simulink library "PTOSim_Lib"  (R2014a)
settings: Solver=ode45  StartTime=0.0  StopTime=10.0  RelTol=1e-3
undefined symbols (not defined in the file): alpha, Amax, Amin, Ap, Beta_e, bf, bg, Cd, D, driveEff, J, k1, k2, omegaBase, omegaInit, pAeq, pAi, pAupper_limit, pBeq, pBi, pBupper_limit, pCprecharge, pDprecharge, pMax, pMin, rho, TgenBase, tot, VC0, VCeq, VD0, VDeq, Vo
settings Model: ForwardingTableString=||__slOldName__||Y:\MATLAB\PTO-Sim\Source\lib||__slNewName__||Y:\MATLAB\PTO-Sim\PassiveHydraulicPTO  Creator=sor  LastModifiedBy=sor

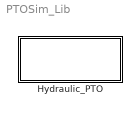
== system PTOSim_Lib ==
  Hydraulic_PTO : Subsystem  RequirementInfo={} %GIDa_f12a42eb_b9cb_4818_b573_b7dee4183a3b

== system PTOSim_Lib/Hydraulic_PTO ==
  Accumulator : Subsystem  Variant=on  mask{pto=0}
      mask prompts: pto "PTO Name"
  Gen Drive Efficiency : Subsystem  mask{pto=0}
      mask prompts: pto "PTO Name"
  "Motor " : Subsystem  mask{pto=0}
      mask prompts: pto "PTO Name"
  "Piston " : Subsystem  mask{pto=0}
      mask prompts: pto "PTO Name"
  Rectified Valve : Subsystem  mask{pto=0}
      mask prompts: pto "PTO Name"

== system PTOSim_Lib/Hydraulic_PTO/Accumulator ==
  note: 1) Only subsystems can be added as variant choices at this level
      | 2) Blocks cannot be connected at this level as connectivity is
      | automatically determined at simulation, based on the active variant
  Vdot : Inport
  Vdotm : Inport  Port=2
  High Pressure Accumulator : Subsystem  VariantControl=Variant
  Low Pressure Accumulator : Subsystem  VariantControl=Variant1
  Pressure : Outport

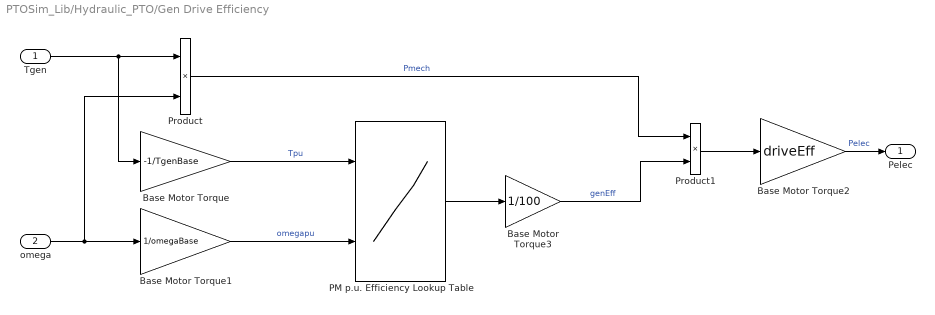
== system PTOSim_Lib/Hydraulic_PTO/Gen Drive Efficiency ==
  Tgen : Inport
  omega : Inport  Port=2
  Base Motor Torque : Gain  Gain=-1/TgenBase
  Base Motor Torque1 : Gain  Gain=1/omegaBase
  Base Motor Torque2 : Gain  Gain=driveEff
  Base Motor Torque3 : Gain  Gain=1/100
  PM p.u. Efficiency Lookup Table : Lookup_n-D  BreakpointsForDimension1=tot.Tpu(:,1)  BreakpointsForDimension2=tot.omegapu(1,:)  Table=tot.eff  InterpMethod=Flat  InputSameDT=on
  Product : Product  RndMeth=Zero
  Product1 : Product  RndMeth=Zero
  Pelec : Outport
  wires:
  Base Motor Torque2/1 -> Pelec/1  "Pelec"
  Product1/1 -> Base Motor Torque2/1
  Product/1 -> Product1/1  "Pmech"
  Base Motor Torque3/1 -> Product1/2  "genEff"
  PM p.u. Efficiency Lookup Table/1 -> Base Motor Torque3/1
  omega/1 -> Product/2, Base Motor Torque1/1
  Base Motor Torque1/1 -> PM p.u. Efficiency Lookup Table/2  "omegapu"
  Tgen/1 -> Base Motor Torque/1, Product/1
  Base Motor Torque/1 -> PM p.u. Efficiency Lookup Table/1  "Tpu"

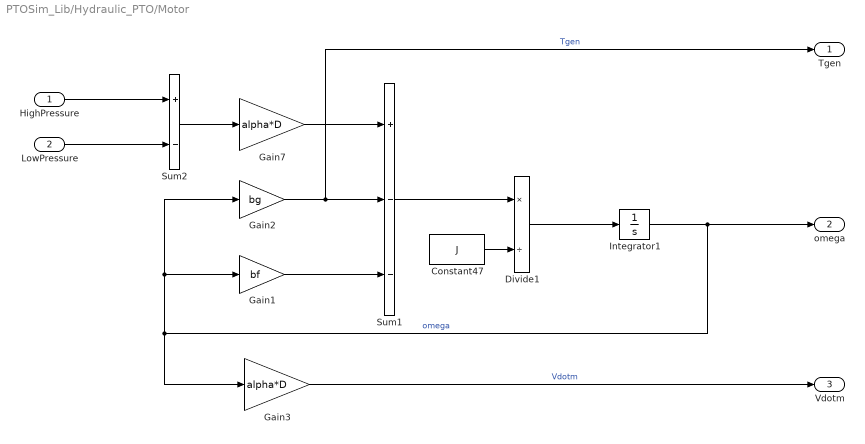
== system PTOSim_Lib/Hydraulic_PTO/Motor  ==
  HighPressure : Inport
  LowPressure : Inport  Port=2
  Constant47 : Constant  Value=J
  Divide1 : Product  Inputs=*/
  Gain1 : Gain  Gain=bf
  Gain2 : Gain  Gain=bg
  Gain3 : Gain  Gain=alpha*D
  Gain7 : Gain  Gain=alpha*D
  Integrator1 : Integrator  InitialCondition=omegaInit
  Sum1 : Sum  Inputs=+--
  Sum2 : Sum  Inputs=+-
  Tgen : Outport
  omega : Outport  Port=2
  Vdotm : Outport  Port=3
  wires:
  Gain7/1 -> Sum1/1
  Gain2/1 -> Tgen/1, Sum1/2  "Tgen"
  Gain1/1 -> Sum1/3
  Sum1/1 -> Divide1/1
  Constant47/1 -> Divide1/2
  Divide1/1 -> Integrator1/1
  Integrator1/1 -> omega/1, Gain3/1, Gain1/1, Gain2/1  "omega"
  Gain3/1 -> Vdotm/1  "Vdotm"
  HighPressure/1 -> Sum2/1
  LowPressure/1 -> Sum2/2
  Sum2/1 -> Gain7/1

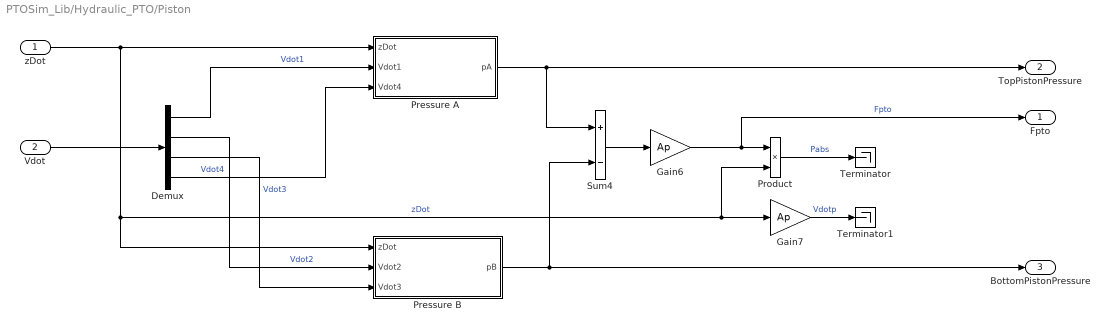
== system PTOSim_Lib/Hydraulic_PTO/Piston  ==
  zDot : Inport
  Vdot : Inport  Port=2
  Demux : Demux
  Gain6 : Gain  Gain=Ap
  Gain7 : Gain  Gain=Ap
  Pressure A : Subsystem
  Pressure B : Subsystem
  Product : Product
  Sum4 : Sum  Inputs=+-
  Terminator : Terminator
  Terminator1 : Terminator
  Fpto : Outport
  TopPistonPressure : Outport  Port=2
  BottomPistonPressure : Outport  Port=3
  wires:
  Pressure A/1(pA) -> Sum4/1, TopPistonPressure/1
  Pressure B/1(pB) -> BottomPistonPressure/1, Sum4/2
  Gain7/1 -> Terminator1/1  "Vdotp"
  Gain6/1 -> Fpto/1, Product/1  "Fpto"
  Product/1 -> Terminator/1  "Pabs"
  Vdot/1 -> Demux/1
  zDot/1 -> Gain7/1, Product/2, Pressure B/1(zDot), Pressure A/1(zDot)  "zDot"
  Demux/1 -> Pressure A/2(Vdot1)  "Vdot1"
  Demux/2 -> Pressure B/2(Vdot2)  "Vdot2"
  Demux/3 -> Pressure B/3(Vdot3)  "Vdot3"
  Demux/4 -> Pressure A/3(Vdot4)  "Vdot4"
  Sum4/1 -> Gain6/1

== system PTOSim_Lib/Hydraulic_PTO/Rectified Valve ==
  TopPistonPressure : Inport
  BottomPistonPressure : Inport  Port=2
  HighPressure : Inport  Port=3
  LowPressure : Inport  Port=4
  Bus Creator : BusCreator
  Subsystem : Subsystem
  Subsystem1 : Subsystem
  Subsystem2 : Subsystem
  Subsystem3 : Subsystem
  Vdot : Outport
  wires:
  TopPistonPressure/1 -> Subsystem3/2(pA), Subsystem/1(pA)
  BottomPistonPressure/1 -> Subsystem2/2(pB), Subsystem1/1(pB)
  HighPressure/1 -> Subsystem1/2(pC), Subsystem/2(pC)
  LowPressure/1 -> Subsystem3/1(pD), Subsystem2/1(pD)
  Subsystem3/1(Vdot4) -> Bus Creator/4  "Vdot4"
  Subsystem2/1(Vdot3) -> Bus Creator/3  "Vdot3"
  Subsystem1/1(Vdot2) -> Bus Creator/2  "Vdot2"
  Subsystem/1(Vdot1) -> Bus Creator/1  "Vdot1"
  Bus Creator/1 -> Vdot/1

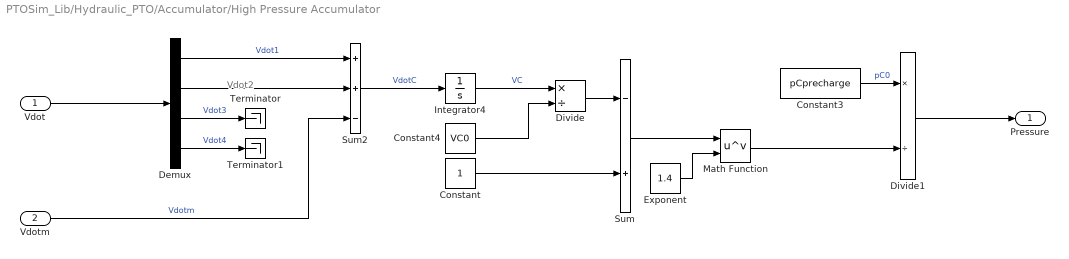
== system PTOSim_Lib/Hydraulic_PTO/Accumulator/High Pressure Accumulator ==
  note: Vdot2
  Vdot : Inport
  Vdotm : Inport  Port=2
  Constant : Constant
  Constant3 : Constant  Value=pCprecharge
  Constant4 : Constant  Value=VC0
  Demux : Demux
  Divide : Product  Inputs=*/
  Divide1 : Product  Inputs=*/
  Exponent : Constant  Value=1.4
  Integrator4 : Integrator  InitialCondition=VCeq
  Math Function : Math  Operator=pow  SaturateOnIntegerOverflow=on
  Sum : Sum  Inputs=-+
  Sum2 : Sum  Inputs=++-
  Terminator : Terminator
  Terminator1 : Terminator
  Pressure : Outport
  wires:
  Sum2/1 -> Integrator4/1  "VdotC"
  Integrator4/1 -> Divide/1  "VC"
  Constant4/1 -> Divide/2
  Constant/1 -> Sum/2
  Divide/1 -> Sum/1
  Exponent/1 -> Math Function/2
  Sum/1 -> Math Function/1
  Math Function/1 -> Divide1/2
  Constant3/1 -> Divide1/1  "pC0"
  Divide1/1 -> Pressure/1
  Vdot/1 -> Demux/1
  Demux/3 -> Terminator/1  "Vdot3"
  Demux/4 -> Terminator1/1  "Vdot4"
  Demux/1 -> Sum2/1  "Vdot1"
  Demux/2 -> Sum2/2
  Vdotm/1 -> Sum2/3  "Vdotm"

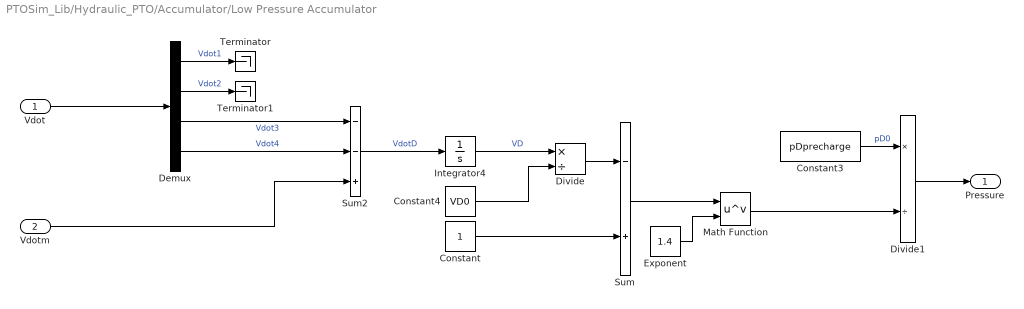
== system PTOSim_Lib/Hydraulic_PTO/Accumulator/Low Pressure Accumulator ==
  Vdot : Inport
  Vdotm : Inport  Port=2
  Constant : Constant
  Constant3 : Constant  Value=pDprecharge
  Constant4 : Constant  Value=VD0
  Demux : Demux
  Divide : Product  Inputs=*/
  Divide1 : Product  Inputs=*/
  Exponent : Constant  Value=1.4
  Integrator4 : Integrator  InitialCondition=VDeq
  Math Function : Math  Operator=pow  SaturateOnIntegerOverflow=on
  Sum : Sum  Inputs=-+
  Sum2 : Sum  Inputs=--+
  Terminator : Terminator
  Terminator1 : Terminator
  Pressure : Outport
  wires:
  Sum2/1 -> Integrator4/1  "VdotD"
  Integrator4/1 -> Divide/1  "VD"
  Constant4/1 -> Divide/2
  Constant/1 -> Sum/2
  Divide/1 -> Sum/1
  Exponent/1 -> Math Function/2
  Sum/1 -> Math Function/1
  Math Function/1 -> Divide1/2
  Constant3/1 -> Divide1/1  "pD0"
  Divide1/1 -> Pressure/1
  Vdot/1 -> Demux/1
  Demux/3 -> Sum2/1  "Vdot3"
  Demux/4 -> Sum2/2  "Vdot4"
  Vdotm/1 -> Sum2/3
  Demux/1 -> Terminator/1  "Vdot1"
  Demux/2 -> Terminator1/1  "Vdot2"

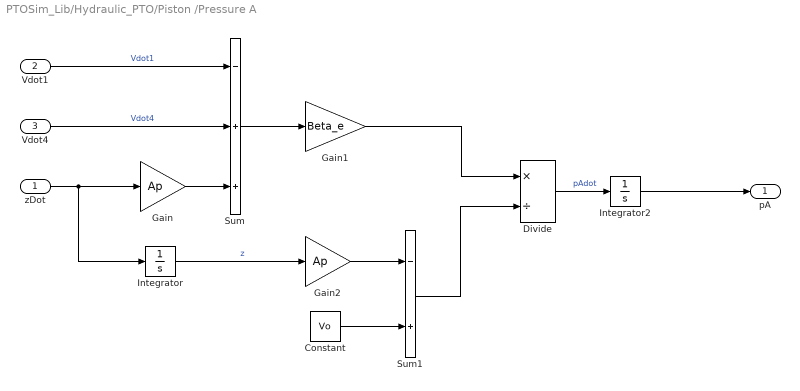
== system PTOSim_Lib/Hydraulic_PTO/Piston /Pressure A ==
  zDot : Inport
  Vdot1 : Inport  Port=2
  Vdot4 : Inport  Port=3
  Constant : Constant  Value=Vo
  Divide : Product  Inputs=*/
  Gain : Gain  Gain=Ap
  Gain1 : Gain  Gain=Beta_e
  Gain2 : Gain  Gain=Ap
  Integrator : Integrator
  Integrator2 : Integrator  InitialCondition=pAi  UpperSaturationLimit=pAupper_limit  LowerSaturationLimit=pAeq
  Sum : Sum  Inputs=-++
  Sum1 : Sum  Inputs=-+
  pA : Outport
  wires:
  Gain/1 -> Sum/3
  Sum/1 -> Gain1/1
  zDot/1 -> Integrator/1, Gain/1
  Integrator/1 -> Gain2/1  "z"
  Gain2/1 -> Sum1/1
  Constant/1 -> Sum1/2
  Gain1/1 -> Divide/1
  Sum1/1 -> Divide/2
  Vdot1/1 -> Sum/1  "Vdot1"
  Divide/1 -> Integrator2/1  "pAdot"
  Vdot4/1 -> Sum/2  "Vdot4"
  Integrator2/1 -> pA/1

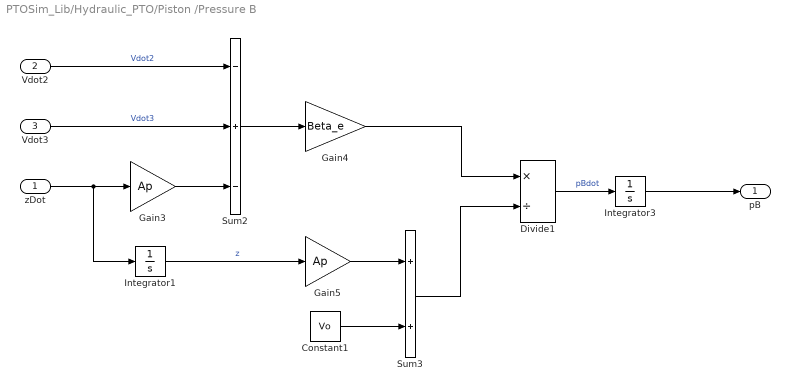
== system PTOSim_Lib/Hydraulic_PTO/Piston /Pressure B ==
  zDot : Inport
  Vdot2 : Inport  Port=2
  Vdot3 : Inport  Port=3
  Constant1 : Constant  Value=Vo
  Divide1 : Product  Inputs=*/
  Gain3 : Gain  Gain=Ap
  Gain4 : Gain  Gain=Beta_e
  Gain5 : Gain  Gain=Ap
  Integrator1 : Integrator
  Integrator3 : Integrator  InitialCondition=pBi  UpperSaturationLimit=pBupper_limit  LowerSaturationLimit=pBeq
  Sum2 : Sum  Inputs=-+-
  Sum3 : Sum
  pB : Outport
  wires:
  Gain3/1 -> Sum2/3
  Sum2/1 -> Gain4/1
  zDot/1 -> Integrator1/1, Gain3/1
  Integrator1/1 -> Gain5/1  "z"
  Gain5/1 -> Sum3/1
  Constant1/1 -> Sum3/2
  Gain4/1 -> Divide1/1
  Sum3/1 -> Divide1/2
  Divide1/1 -> Integrator3/1  "pBdot"
  Vdot2/1 -> Sum2/1  "Vdot2"
  Vdot3/1 -> Sum2/2  "Vdot3"
  Integrator3/1 -> pB/1

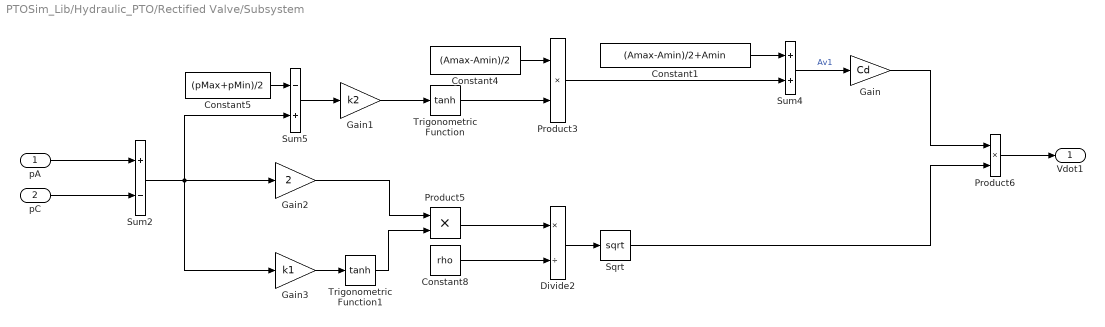
== system PTOSim_Lib/Hydraulic_PTO/Rectified Valve/Subsystem ==
  pA : Inport
  pC : Inport  Port=2
  Constant1 : Constant  Value=(Amax-Amin)/2+Amin
  Constant4 : Constant  Value=(Amax-Amin)/2
  Constant5 : Constant  Value=(pMax+pMin)/2
  Constant8 : Constant  Value=rho
  Divide2 : Product  Inputs=*/
  Gain : Gain  Gain=Cd
  Gain1 : Gain  Gain=k2
  Gain2 : Gain  Gain=2
  Gain3 : Gain  Gain=k1
  Product3 : Product
  Product5 : Product
  Product6 : Product
  Sqrt : Sqrt  SaturateOnIntegerOverflow=on
  Sum2 : Sum  Inputs=+-
  Sum4 : Sum
  Sum5 : Sum  Inputs=-+
  Trigonometric Function : Trigonometry  Operator=tanh
  Trigonometric Function1 : Trigonometry  Operator=tanh
  Vdot1 : Outport
  wires:
  Gain1/1 -> Trigonometric Function/1
  Trigonometric Function/1 -> Product3/2
  Product3/1 -> Sum4/2
  Sum5/1 -> Gain1/1
  Sum4/1 -> Gain/1  "Av1"
  Gain3/1 -> Trigonometric Function1/1
  Gain2/1 -> Product5/1
  Trigonometric Function1/1 -> Product5/2
  Sqrt/1 -> Product6/2
  Gain/1 -> Product6/1
  Constant8/1 -> Divide2/2
  Product5/1 -> Divide2/1
  Divide2/1 -> Sqrt/1
  pA/1 -> Sum2/1
  pC/1 -> Sum2/2
  Product6/1 -> Vdot1/1
  Constant4/1 -> Product3/1
  Constant5/1 -> Sum5/1
  Constant1/1 -> Sum4/1
  Sum2/1 -> Gain3/1, Sum5/2, Gain2/1

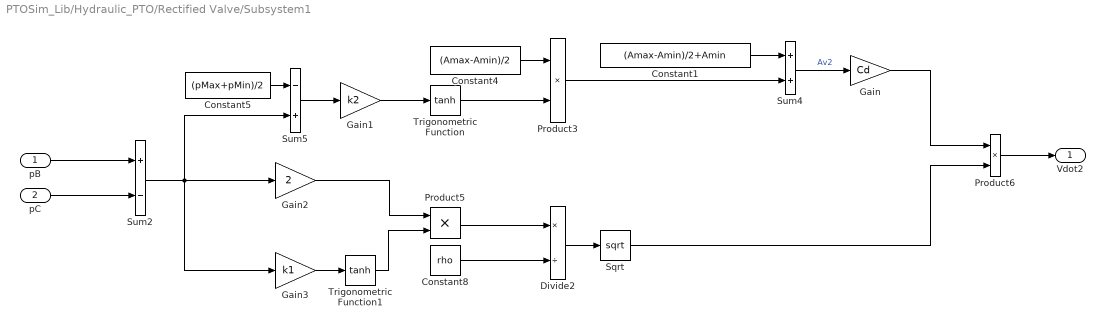
== system PTOSim_Lib/Hydraulic_PTO/Rectified Valve/Subsystem1 ==
  pB : Inport
  pC : Inport  Port=2
  Constant1 : Constant  Value=(Amax-Amin)/2+Amin
  Constant4 : Constant  Value=(Amax-Amin)/2
  Constant5 : Constant  Value=(pMax+pMin)/2
  Constant8 : Constant  Value=rho
  Divide2 : Product  Inputs=*/
  Gain : Gain  Gain=Cd
  Gain1 : Gain  Gain=k2
  Gain2 : Gain  Gain=2
  Gain3 : Gain  Gain=k1
  Product3 : Product
  Product5 : Product
  Product6 : Product
  Sqrt : Sqrt  SaturateOnIntegerOverflow=on
  Sum2 : Sum  Inputs=+-
  Sum4 : Sum
  Sum5 : Sum  Inputs=-+
  Trigonometric Function : Trigonometry  Operator=tanh
  Trigonometric Function1 : Trigonometry  Operator=tanh
  Vdot2 : Outport
  wires:
  Gain1/1 -> Trigonometric Function/1
  Trigonometric Function/1 -> Product3/2
  Product3/1 -> Sum4/2
  Sum5/1 -> Gain1/1
  Sum4/1 -> Gain/1  "Av2"
  Gain3/1 -> Trigonometric Function1/1
  Gain2/1 -> Product5/1
  Trigonometric Function1/1 -> Product5/2
  Sqrt/1 -> Product6/2
  Gain/1 -> Product6/1
  Constant8/1 -> Divide2/2
  Product5/1 -> Divide2/1
  Divide2/1 -> Sqrt/1
  pB/1 -> Sum2/1
  pC/1 -> Sum2/2
  Product6/1 -> Vdot2/1
  Constant4/1 -> Product3/1
  Constant5/1 -> Sum5/1
  Constant1/1 -> Sum4/1
  Sum2/1 -> Gain3/1, Sum5/2, Gain2/1

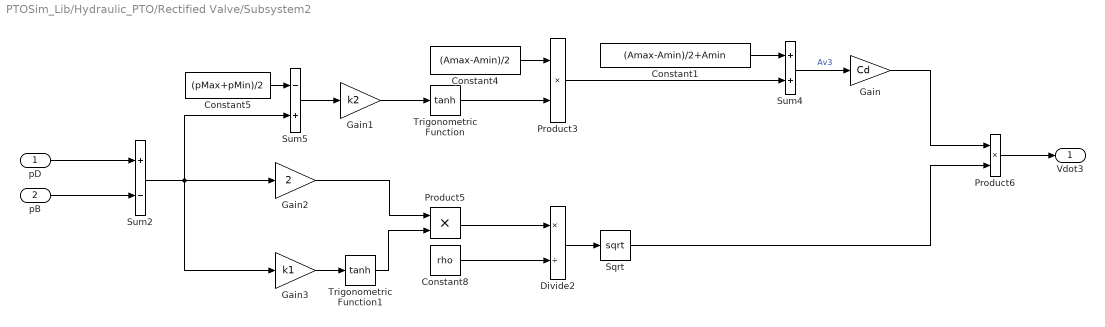
== system PTOSim_Lib/Hydraulic_PTO/Rectified Valve/Subsystem2 ==
  pD : Inport
  pB : Inport  Port=2
  Constant1 : Constant  Value=(Amax-Amin)/2+Amin
  Constant4 : Constant  Value=(Amax-Amin)/2
  Constant5 : Constant  Value=(pMax+pMin)/2
  Constant8 : Constant  Value=rho
  Divide2 : Product  Inputs=*/
  Gain : Gain  Gain=Cd
  Gain1 : Gain  Gain=k2
  Gain2 : Gain  Gain=2
  Gain3 : Gain  Gain=k1
  Product3 : Product
  Product5 : Product
  Product6 : Product
  Sqrt : Sqrt  SaturateOnIntegerOverflow=on
  Sum2 : Sum  Inputs=+-
  Sum4 : Sum
  Sum5 : Sum  Inputs=-+
  Trigonometric Function : Trigonometry  Operator=tanh
  Trigonometric Function1 : Trigonometry  Operator=tanh
  Vdot3 : Outport
  wires:
  Gain1/1 -> Trigonometric Function/1
  Trigonometric Function/1 -> Product3/2
  Product3/1 -> Sum4/2
  Sum5/1 -> Gain1/1
  Sum4/1 -> Gain/1  "Av3"
  Gain3/1 -> Trigonometric Function1/1
  Gain2/1 -> Product5/1
  Trigonometric Function1/1 -> Product5/2
  Sqrt/1 -> Product6/2
  Gain/1 -> Product6/1
  Constant8/1 -> Divide2/2
  Product5/1 -> Divide2/1
  Divide2/1 -> Sqrt/1
  pD/1 -> Sum2/1
  pB/1 -> Sum2/2
  Product6/1 -> Vdot3/1
  Constant4/1 -> Product3/1
  Constant5/1 -> Sum5/1
  Constant1/1 -> Sum4/1
  Sum2/1 -> Gain3/1, Sum5/2, Gain2/1

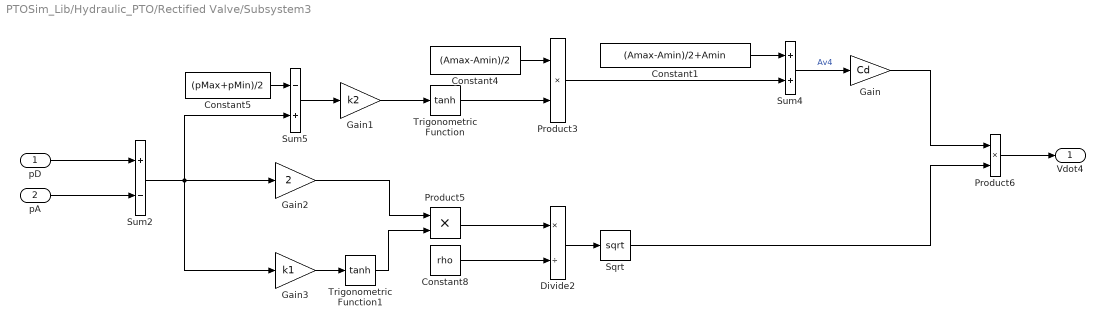
== system PTOSim_Lib/Hydraulic_PTO/Rectified Valve/Subsystem3 ==
  pD : Inport
  pA : Inport  Port=2
  Constant1 : Constant  Value=(Amax-Amin)/2+Amin
  Constant4 : Constant  Value=(Amax-Amin)/2
  Constant5 : Constant  Value=(pMax+pMin)/2
  Constant8 : Constant  Value=rho
  Divide2 : Product  Inputs=*/
  Gain : Gain  Gain=Cd
  Gain1 : Gain  Gain=k2
  Gain2 : Gain  Gain=2
  Gain3 : Gain  Gain=k1
  Product3 : Product
  Product5 : Product
  Product6 : Product
  Sqrt : Sqrt  SaturateOnIntegerOverflow=on
  Sum2 : Sum  Inputs=+-
  Sum4 : Sum
  Sum5 : Sum  Inputs=-+
  Trigonometric Function : Trigonometry  Operator=tanh
  Trigonometric Function1 : Trigonometry  Operator=tanh
  Vdot4 : Outport
  wires:
  Gain1/1 -> Trigonometric Function/1
  Trigonometric Function/1 -> Product3/2
  Product3/1 -> Sum4/2
  Sum5/1 -> Gain1/1
  Sum4/1 -> Gain/1  "Av4"
  Gain3/1 -> Trigonometric Function1/1
  Gain2/1 -> Product5/1
  Trigonometric Function1/1 -> Product5/2
  Sqrt/1 -> Product6/2
  Gain/1 -> Product6/1
  Constant8/1 -> Divide2/2
  Product5/1 -> Divide2/1
  Divide2/1 -> Sqrt/1
  pD/1 -> Sum2/1
  pA/1 -> Sum2/2
  Product6/1 -> Vdot4/1
  Constant4/1 -> Product3/1
  Constant5/1 -> Sum5/1
  Constant1/1 -> Sum4/1
  Sum2/1 -> Gain3/1, Sum5/2, Gain2/1
